simulink model "Quadruped"  (R2020a)
settings: Solver=VariableStepAuto  StartTime=0.0  StopTime=10.0  RelTol=1e-3  EnableMultiTasking=on
PreLoadFcn:
  | Parameters;
values from neighbouring files (symbols this model uses):
  buffer = 8000    [Parameters.m]
  gait_time = 1    [Parameters.m]
  l1 = 0.2    [Parameters.m]
  l2 = 0.4    [Parameters.m]
  l3 = l3_orig-r    (= 0.38)    [Parameters.m]
  robot_b = 0.1    [Parameters.m]
  robot_l = 1    [Parameters.m]
  robot_w = 0.4    [Parameters.m]
  step_height = 0.1    [Parameters.m]
  step_time = gait_time/2    (= 0.5)    [Parameters.m]
  target1 = 0    [Parameters.m]
  target2 = 30    [Parameters.m]
  target2r = -30    [Parameters.m]
  target3 = -120    [Parameters.m]
  target3r = 120    [Parameters.m]
  Xc_i = 0    [Parameters.m]
undefined symbols (not defined in the file or in its folder): X, Y, Z
libraries: sm_lib x76, nesl_utility x46, simulink x26
(part 4 of 4)

== matlab function Quadruped/Motor Inputs/Inverse Kinematics/IK L ==
  data: x input; theta1 output; y input; z input; theta2 output; theta3 output
function [theta1,theta2,theta3] = IK(x,y,z)
% (x,y,z) in hip frame of each leg
% Write equations of each angle
l1 = 0.2;
l2 = 0.4;
l3 = 0.4;
brute_error = 3;
c = sqrt((x-l1)^2 + z^2);
theta3 = acosd((l2^2 + l3^2 - c^2)/(2*l2*l3)) - 180;
beta = acosd((c^2 + l2^2 - l3^2)/(2*l2*c));
theta2 = atand(((c*sind(beta)-l3*sind(theta3))/(l3*cosd(theta3)+c*cosd(beta)-l2)))+ brute_error;
theta1 = atand(y/(l1+l2*cos(theta2)+l3*cos(theta3)));

% t1 range [-90,90] here also true in atand and in actual bot never to violate this range
% t2 range [-90,90] here also true in atand and in actual bot never to violate this range
% t3 range [0,180] here true in acosd and in actual bot for left leg [-180,0]
% t3 range can be increased to [-180,180] for giving capability for legs to do task

== matlab function Quadruped/Motor Inputs/Inverse Kinematics/IK R 1 ==
  data: x input; theta1 output; y input; z input; theta2 output; theta3 output
function [theta1,theta2,theta3] = IK(x,y,z)
% (x,y,z) in hip frame of each leg
% Write equations of each angle
l1 = 0.2;
l2 = 0.4;
l3 = 0.4;
brute_error = 3;
c = sqrt((x-l1)^2 + z^2);
theta3 = acosd((l2^2 + l3^2 - c^2)/(2*l2*l3));
beta = acosd((c^2 + l2^2 - l3^2)/(2*l2*c));
theta2 = atand(((c*sind(beta)-l3*sind(theta3))/(l3*cosd(theta3)+c*cosd(beta)-l2)))+ brute_error;
theta1 = atand(y/(l1+l2*cos(theta2)+l3*cos(theta3)));

% t1 range [-90,90] here also true in atand and in actual bot never to violate this range
% t2 range [-90,90] here also true in atand and in actual bot never to violate this range
% t3 range [0,180] here true in acosd and in actual bot for right leg true
% t3 range can be increased to [-180,180] for giving capability for legs to do task

== matlab function Quadruped/Motor Inputs/Inverse Kinematics/Transform to BR Hip ==
  data: x input; X output; y input; z input; Y output; Z output
function [X,Y,Z] = WorldToBR(x,y,z)
% (x,y,z) input in World frame
% [X,Y,Z] output in Right legs Hip frame

%Define T transformation matrix
robot_w = 0.4;
robot_l = 1;
h = 0.25;
T = [0 1 0 -robot_w/2;
    -1 0 0 robot_l/2;
    0 0 1 -h;
    0 0 0 1];

wf = [x; y; z; 1];

hf = T*wf;

X = hf(1,1);
Y = hf(2,1);
Z = hf(3,1);
